simulink model "EX_Case_1"  (Simulink 4.00)
settings: Solver=ode45  StartTime=0.0  StopTime=1  MaxStep=0.01  RelTol=1e-3

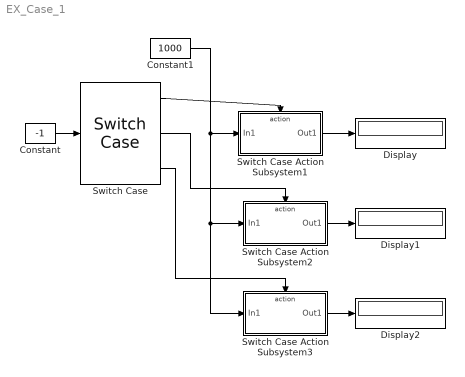
== system EX_Case_1 ==
  Constant : Constant  Value=-1
  Constant1 : Constant  Value=1000
  Display : Display
      settings: Format=short
  Display1 : Display
      settings: Format=short
  Display2 : Display
      settings: Format=short
  Switch Case : SwitchCase  CaseConditions={1, -1}  CaseShowDefault=on
  Switch Case Action Subsystem1 : Subsystem  TreatAsAtomicUnit=on
      settings: RTWFcnNameOpts=Auto  RTWFileNameOpts=Auto
  Switch Case Action Subsystem2 : Subsystem  TreatAsAtomicUnit=on
      settings: RTWFcnNameOpts=Auto  RTWFileNameOpts=Auto
  Switch Case Action Subsystem3 : Subsystem  TreatAsAtomicUnit=on
      settings: RTWFcnNameOpts=Auto  RTWFileNameOpts=Auto
  wires:
  Switch Case/1 -> Switch Case Action Subsystem1/Action
  Constant/1 -> Switch Case/1
  Switch Case Action Subsystem1/1(Out1) -> Display/1
  Constant1/1 -> Switch Case Action Subsystem2/1(In1), Switch Case Action Subsystem3/1(In1), Switch Case Action Subsystem1/1(In1)
  Switch Case Action Subsystem2/1(Out1) -> Display1/1
  Switch Case Action Subsystem3/1(Out1) -> Display2/1
  Switch Case/2 -> Switch Case Action Subsystem2/Action
  Switch Case/3 -> Switch Case Action Subsystem3/Action

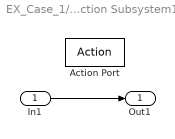
== system EX_Case_1/Switch Case Action Subsystem1 ==
  In1 : Inport  Port=1  LatchInput=off
  Action Port : ActionPort  InitializeStates=held  ActionType=case
  Out1 : Outport  Port=1
  wires:
  In1/1 -> Out1/1

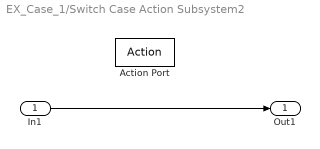
== system EX_Case_1/Switch Case Action Subsystem2 ==
  In1 : Inport  Port=1  LatchInput=off
  Action Port : ActionPort  InitializeStates=held  ActionType=case
  Out1 : Outport  Port=1
  wires:
  In1/1 -> Out1/1

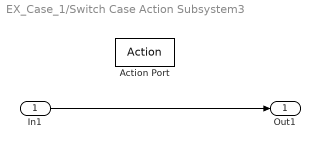
== system EX_Case_1/Switch Case Action Subsystem3 ==
  In1 : Inport  Port=1  LatchInput=off
  Action Port : ActionPort  InitializeStates=held  ActionType=default
  Out1 : Outport  Port=1
  wires:
  In1/1 -> Out1/1
